simulink library "Copter_Library"  (Simulink 7.5)
settings: Solver=ode45  StartTime=0.0  StopTime=10.0  RelTol=1e-3
values from neighbouring files (symbols this model uses):
  phi0 = 0.15    [Quadrocopter_control_Driver.m]    (also in calc_stability.m = 0)
  r_phi0 = 0    [Quadrocopter_control_Driver.m]    (also in calc_stability.m)
  r_psi0 = 0    [Quadrocopter_control_Driver.m]    (also in calc_stability.m)
  r_theta0 = 0    [Quadrocopter_control_Driver.m]    (also in calc_stability.m)
  theta0 = 0.15    [Quadrocopter_control_Driver.m]    (also in calc_stability.m = 0)
  Ts = 0.01    [Reglerauslegung.m]    (also in Test_Reglerauslegung.m)
undefined symbols (not defined in the file or in its folder): boom, DiscIntNeverNeededParam, f1, f2, f3, f4, f5, g, I_x, I_y, I_z, m, speed, thrust, Ts_Opt
libraries: simulink x21, Copter_Library x17, vrlib x7, dspobslib x4, dspinverses x3, Control_lib x2
(part 1 of 3)
settings Model: Creator=robert  LastModifiedBy=Anonymos

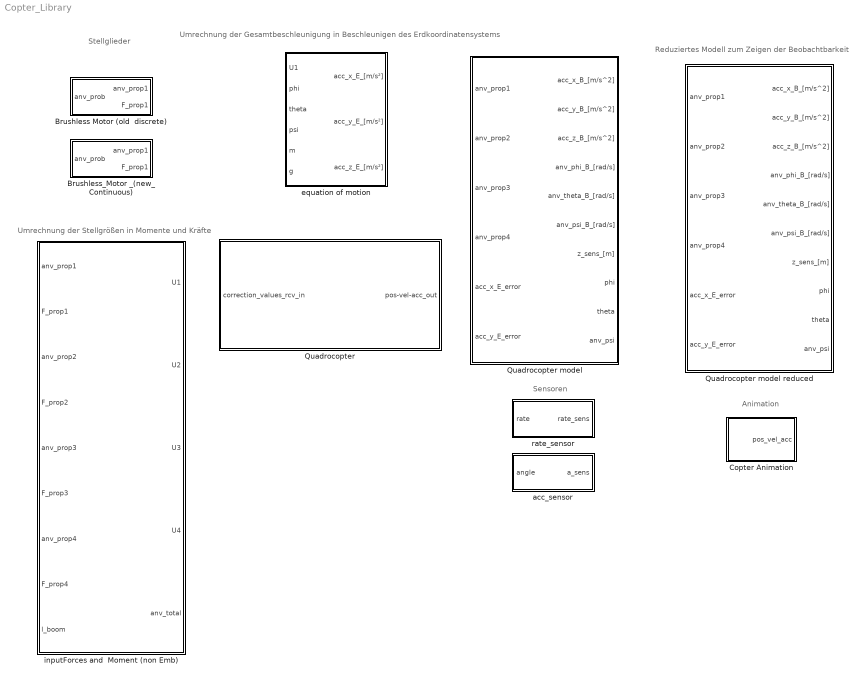
== system Copter_Library ==
  note: Sensoren
  note: Animation
  note: Umrechnung der Gesamtbeschleunigung in
      | Beschleunigen des Erdkoordinatensystems
  note: Stellglieder
  note: Umrechnung der Stellgrößen
      | in Momente und Kräfte
  note: Reduziertes Modell zum Zeigen der
      | Beobachtbarkeit
  Brushless Motor (old  discrete) : Subsystem
  Brushless_Motor _(new_Continuous) : Subsystem  mask{M_error=0.99}
      mask prompts: M_error "Motor-Force pitch error [1 = no error, 0.9 = 10% negativ error, 1.1 = 10% positive error]:"
  Copter Animation : Subsystem  mask(Quadrocopter Animation){AXES=[-100 100 -100 100 0 100], T_INT=1/25, K_VAR=Feste Position, K_POS=[10 0 2], K_ANGLE=27, A_ON=on, u_phi=on, u_theta=on, u_psi=on, u_x=on, u_y=on, u_z=off}
      mask prompts: AXES "Achsen Grenzen [xmin xmax ymin ymax zmin zmax]"; T_INT "Zeitintervall zwischen Aktualisierungen [s]:"; K_VAR "Kamera Art:"; K_POS "Ort der Kamera [xc yc zc]:"; K_ANGLE "Öffnungswinkel der Kamera [Grad]:"; A_ON "Animation Einschalten:"; u_phi "Use Input phi:"; u_theta "Use Input theta:"; u_psi "Use Input psi:"; u_x "Use Input x:"; u_y "Use Input y:"; u_z "Use Input z:"
      mask help: Erstellt eine 3-D animierte Ansicht eines Quadrocopters.
      mask init:
      | Config.axes = AXES;
      | Config.update = T_INT;
      | Config.camera_view = K_VAR;
      | Config.camera_pos = K_POS;
      | Config.view = K_ANGLE;
      | Config.Animenable = A_ON;
      | Config.phi = u_phi;
      | Config.theta = u_theta;
      | Config.psi = u_psi;
      | Config.x = u_x;
      | Config.y = u_y;
      | Config.z = u_z;
      mask Help:
      | <p>Dieser Block erstellt ein 3 dimensionales Fenster eines Quadrocopters.
      | 
      | <p><H4>Block Eingänge</H4>
      | Der Eingangsvektor bestehend aus:
      | <ul>
      | <li>X-Koordinate - Ort bezogen auf die X-Achse
      | <li>Y-Koordinate - Ort bezogen auf die Y-Achse
      | <li>Z-Koordinate - Ort bezogen auf die Z-Achse
      | <li>Psi - Yaw Drehung um die Z-Achse
      | <li>Phi - Roll Drehen um die Achse in Flugrichtung
      | <li>theta - pitch Neigung in Flugrichtung nach oben bzw. unten
      | </ul></p>
      mask StyleString: edit,edit,popup(Feste Position|Frei bewegbar),edit,edit,checkbox,checkbox,checkbox,checkbox,checkbox,checkbox,checkbox
  Quadrocopter : Subsystem
  Quadrocopter model : Subsystem
  Quadrocopter model reduced : Subsystem
  acc_sensor : Subsystem  mask{lsb_per_g=g/340, direction=1}
      mask prompts: lsb_per_g "Auflösung[LSB/g]:(g = Erdbeschleunigung)"; direction "Direction[-1 ... 1]:"
      mask init:
      | LSB_per_g = lsb_per_g;
      | Direction = direction;
  equation of motion : Subsystem
  inputForces and  Moment (non Emb) : Subsystem
  rate_sensor : Subsystem  mask{resolution=0.01423597337917052316100312926969, offset=505, direction=1}
      mask prompts: resolution "Resolution [(rad/sec)/LSB)]:"; offset "Offset [LSB]:"; direction "Direction [-1 ... 1]"
      mask init:
      | Resolution = resolution;
      | Offset = offset;
      | Direction = direction;

== system Copter_Library/Brushless Motor (old  discrete) ==
  note: Gain of BLDC1
  note: Kraft in Drehzahl umrechnen
  note: Registerwert in Kraft umsetzten
  note: Kraft verzögert, aber Drehzahl nicht ?
  anv_prob : Inport  OutDataType=fixdt(1, 16)  OutScaling=2^0
  Discrete Transfer Fcn : DiscreteTransferFcn  Numerator=[0.05]  Denominator=[1 -0.95]  SampleTime=Ts
  Gain6 : Gain  ParameterDataType=fixdt(1, 16)  ParameterScaling=2^0  OutDataType=fixdt(1, 16)  OutScaling=2^0
  setpoint_thrust_prop1 : Lookup  InputValues=[0 40 175]  Table=[0 500 4500]./1000  LookUpMeth=Interpolation-Use End Values  OutDataType=fixdt(1, 16)  OutScaling=2^0
  thrust_speed_prop1 : Lookup  InputValues=thrust  Table=speed  LookUpMeth=Interpolation-Use End Values  OutDataType=fixdt(1, 16)  OutScaling=2^0
  anv_prop1 : Outport  OutDataType=fixdt(1, 16)  OutScaling=2^0
  F_prop1 : Outport  Port=2  OutDataType=fixdt(1, 16)  OutScaling=2^0
  wires:
  anv_prob/1 -> setpoint_thrust_prop1/1
  Discrete Transfer Fcn/1 -> Gain6/1
  Gain6/1 -> F_prop1/1
  thrust_speed_prop1/1 -> anv_prop1/1
  setpoint_thrust_prop1/1 -> thrust_speed_prop1/1, Discrete Transfer Fcn/1

== system Copter_Library/Brushless_Motor _(new_Continuous) ==
  note: Gain of BLDC
  note: Kraft in Drehzahl umrechnen
  note: Registerwert in Kraft umsetzten
  note: Verrzögerung des Kraft
  note: Brushless Motor (new Continuous)
  anv_prob : Inport  OutDataType=fixdt(1, 16)  OutScaling=2^0
  Data Type Conversion : DataTypeConversion  OutDataTypeMode=double  OutDataType=fixdt(1, 16)  OutScaling=2^0  OutDataTypeStr=double
  Gain6 : Gain  Gain=M_error  ParameterDataType=fixdt(1, 16)  ParameterScaling=2^0  OutDataType=fixdt(1, 16)  OutScaling=2^0
  Motor_Delay : TransferFcn  Denominator=[0.001 1]  ContinuousStateAttributes='Motor_Delay'
  Saturation : Saturate  UpperLimit=255  LowerLimit=0  OutDataType=fixdt(1, 16)  OutScaling=2^0
  setpoint_thrust_prop : Lookup  InputValues=[0 40 175]  Table=[0 500 4500]./1000  LookUpMeth=Interpolation-Use End Values  OutDataType=fixdt(1, 16)  OutScaling=2^0
  thrust_speed_prop : Lookup  InputValues=thrust  Table=speed  LookUpMeth=Interpolation-Use End Values  OutDataType=fixdt(1, 16)  OutScaling=2^0
  anv_prop1 : Outport  OutDataType=fixdt(1, 16)  OutScaling=2^0
  F_prop1 : Outport  Port=2  OutDataType=fixdt(1, 16)  OutScaling=2^0
  wires:
  setpoint_thrust_prop/1 -> Motor_Delay/1
  Saturation/1 -> Data Type Conversion/1
  anv_prob/1 -> Saturation/1
  Data Type Conversion/1 -> setpoint_thrust_prop/1
  Motor_Delay/1 -> Gain6/1
  Gain6/1 -> F_prop1/1, thrust_speed_prop/1
  thrust_speed_prop/1 -> anv_prop1/1

== system Copter_Library/Copter Animation ==
  pos_vel_acc : Inport  PortDimensions=19  OutDataType=sfix(16)  OutScaling=2^0
  S-Function : S-Function  FunctionName=Copter_Animation  Parameters=Config  EnableBusSupport=off
  Selector2 : Selector  InputPortWidth=19  IndexOptions=Index vector (dialog)  Indices=[1 2 3 4 5 6]  OutputSizes=1
  wires:
  Selector2/1 -> S-Function/1
  pos_vel_acc/1 -> Selector2/1

== system Copter_Library/Quadrocopter ==
  note: pos-vel-acc: [x, y, z, phi(roll), theta(pitch), psi(yaw), vx, vy, vz,rphi(roll rate), rtheta(pitch rate), rpsi(yaw rate),ax, ay, az,aphi(roll rate), atheta(pitch rate), apsi(yaw rate)]
  correction_values_rcv_in : Inport
  Analysis Lab : Subsystem
      mask Display: image(imresize(imread('DecoImg/Lab.jpg'),0.12), 'center');
  Control : Subsystem
      mask Display: image(imresize(imread('DecoImg/Control.jpg'),0.2), 'center');
  Dynamics : Subsystem
      mask Display: image(imresize(imread('DecoImg/Dynamics.jpg'),0.2), 'center');
  Environmetal influences : Subsystem
      mask Display: image(imresize(imread('DecoImg/Environment.jpg'),0.2), 'center');
  Remote Control : Subsystem
      mask Display: image(imresize(imread('DecoImg/RemoteControl.jpg'),0.4), 'center');
  Sensors : Subsystem
      mask Display: image(imresize(imread('DecoImg/Sensors.jpg'),0.1), 'center');
  pos-vel-acc_out : Outport
  wires:
  Control/1(Motors) -> Dynamics/2(Motors)
  Dynamics/1(pos-vel-acc) -> Analysis Lab/1(pos-vel-acc_in), Sensors/1(pos-vel-acc), pos-vel-acc_out/1  "pos-vel-acc"
  Sensors/2(IMU) -> Control/3(IMU)  "ax  ay  rphi  rtheta rpsi"
  Remote Control/1(RC_out) -> Control/1(Task)  "phi(roll) theta(pitch) rpsi(yaw rate) T(thrust)"
  Sensors/1(height) -> Control/4(height)  "height"
  Sensors/3(correction) -> Control/2(correction)  "vx vy rpsi"
  Environmetal influences/1(vel_err) -> Dynamics/1(vel_errors)
  correction_values_rcv_in/1 -> Sensors/2(correction_values_rcv)

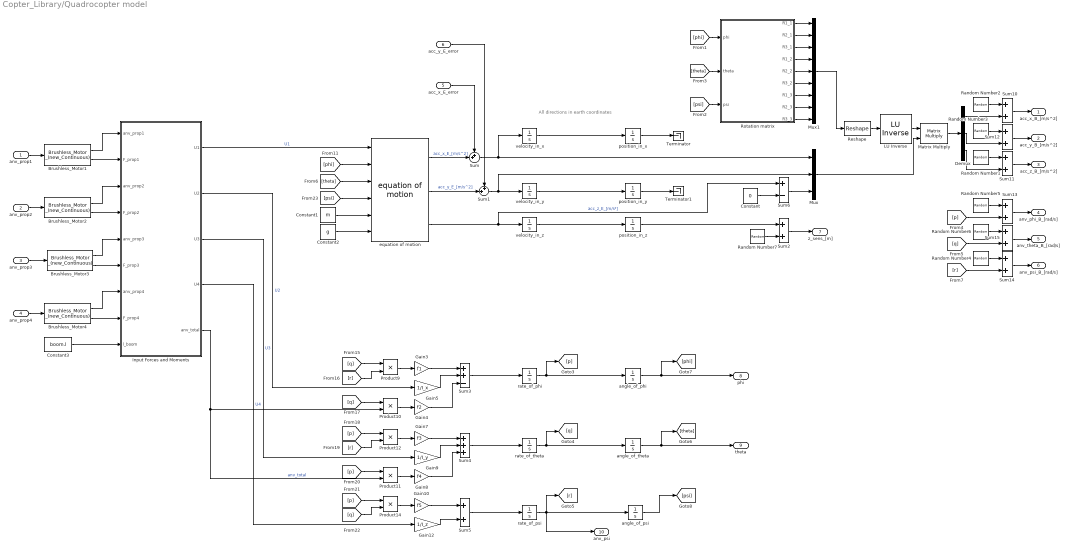
== system Copter_Library/Quadrocopter model ==
  note: All directions in earth coordinates
  anv_prop1 : Inport  OutDataType=fixdt(1, 16)  OutScaling=2^0
  anv_prop2 : Inport  Port=2  OutDataType=fixdt(1, 16)  OutScaling=2^0
  anv_prop3 : Inport  Port=3  OutDataType=fixdt(1, 16)  OutScaling=2^0
  anv_prop4 : Inport  Port=4  OutDataType=fixdt(1, 16)  OutScaling=2^0
  acc_x_E_error : Inport  Port=5  OutDataType=fixdt(1, 16)  OutScaling=2^0
  acc_y_E_error : Inport  Port=6  OutDataType=fixdt(1, 16)  OutScaling=2^0
  " LU Inverse" : dspinverses/ LU Inverse  SystemSampleTime=-1
  Brushless_Motor{1..4} (4 alike) : Copter_Library/Brushless_Motor _(new_Continuous)  SystemSampleTime=-1
  Constant : Constant  Value=0  OutDataType=fixdt(1, 16)  OutScaling=2^0  SampleTime=Ts
  Constant1 : Constant  Value=m  OutDataType=fixdt(1, 16)  OutScaling=2^0  SampleTime=Ts
  Constant2 : Constant  Value=g  OutDataType=fixdt(1, 16)  OutScaling=2^0  SampleTime=Ts
  Constant3 : Constant  Value=boom.l  OutDataType=fixdt(1, 16)  OutScaling=2^0
  Demux : Demux  Outputs=3
  Gain10 : Gain  Gain=f5  ParameterDataType=fixdt(1, 16)  ParameterScaling=2^0  OutDataType=fixdt(1, 16)  OutScaling=2^0
  Gain12 : Gain  Gain=1/I_z  ParameterDataType=fixdt(1, 16)  ParameterScaling=2^0  OutDataType=fixdt(1, 16)  OutScaling=2^0
  Gain3 : Gain  Gain=f1  ParameterDataType=fixdt(1, 16)  ParameterScaling=2^0  OutDataType=fixdt(1, 16)  OutScaling=2^0
  Gain4 : Gain  Gain=f2  ParameterDataType=fixdt(1, 16)  ParameterScaling=2^0  OutDataType=fixdt(1, 16)  OutScaling=2^0
  Gain5 : Gain  Gain=1/I_x  ParameterDataType=fixdt(1, 16)  ParameterScaling=2^0  OutDataType=fixdt(1, 16)  OutScaling=2^0
  Gain7 : Gain  Gain=f3  ParameterDataType=fixdt(1, 16)  ParameterScaling=2^0  OutDataType=fixdt(1, 16)  OutScaling=2^0
  Gain8 : Gain  Gain=f4  ParameterDataType=fixdt(1, 16)  ParameterScaling=2^0  OutDataType=fixdt(1, 16)  OutScaling=2^0
  Gain9 : Gain  Gain=1/I_y  ParameterDataType=fixdt(1, 16)  ParameterScaling=2^0  OutDataType=fixdt(1, 16)  OutScaling=2^0
  Input Forces and Moments : Stateflow chart  TreatAsAtomicUnit=on
  Matrix Multiply : Product  Multiplication=Matrix(*)  OutDataType=sfix(16)  OutScaling=2^0
  Mux : Mux  Inputs=3
  Mux1 : Mux  Inputs=9
  Product{9..12,14} (5 alike) : Product  OutDataType=fixdt(1, 16)  OutScaling=2^0  RndMeth=Zero
  Random Number{1..7} (7 alike) : RandomNumber  Variance=0  SampleTime=Ts
  Reshape : Reshape  OutputDimensionality=Customize  OutputDimensions=[3,3]
  Rotation matrix : Stateflow chart  TreatAsAtomicUnit=on
  Sum : Sum  Inputs=++|  OutDataType=fixdt(1, 16)  OutScaling=2^0
  Sum1 : Sum  Inputs=++|  OutDataType=fixdt(1, 16)  OutScaling=2^0
  Sum{2,5,10..15} (8 alike) : Sum  OutDataType=fixdt(1, 16)  OutScaling=2^0
  Sum3 : Sum  Inputs=++-  OutDataType=fixdt(1, 16)  OutScaling=2^0
  Sum4 : Sum  Inputs=+++  OutDataType=fixdt(1, 16)  OutScaling=2^0
  Sum6 : Sum  Inputs=+-  OutDataType=fixdt(1, 16)  OutScaling=2^0
  Terminator : Terminator
  Terminator1 : Terminator
  angle_of_phi : Integrator
  angle_of_psi : Integrator
  angle_of_theta : Integrator
  equation of motion : Copter_Library/equation of motion  SystemSampleTime=-1
  position_in_x : Integrator
  position_in_y : Integrator
  position_in_z : Integrator
  rate_of_phi : Integrator
  rate_of_psi : Integrator
  rate_of_theta : Integrator
  velocity_in_x : Integrator
  velocity_in_y : Integrator
  velocity_in_z : Integrator
  acc_x_B_[m/s^2] : Outport  OutDataType=fixdt(1, 16)  OutScaling=2^0
  acc_y_B_[m/s^2] : Outport  Port=2  OutDataType=fixdt(1, 16)  OutScaling=2^0
  acc_z_B_[m/s^2] : Outport  Port=3  OutDataType=fixdt(1, 16)  OutScaling=2^0
  anv_phi_B_[rad/s] : Outport  Port=4  OutDataType=fixdt(1, 16)  OutScaling=2^0
  anv_theta_B_[rad/s] : Outport  Port=5  OutDataType=fixdt(1, 16)  OutScaling=2^0
  anv_psi_B_[rad/s] : Outport  Port=6  OutDataType=fixdt(1, 16)  OutScaling=2^0
  z_sens_[m] : Outport  Port=7  OutDataType=fixdt(1, 16)  OutScaling=2^0
  phi : Outport  Port=8  OutDataType=fixdt(1, 16)  OutScaling=2^0
  theta : Outport  Port=9  OutDataType=fixdt(1, 16)  OutScaling=2^0
  anv_psi : Outport  Port=10  OutDataType=fixdt(1, 16)  OutScaling=2^0
  wires:
  Sum14/1 -> anv_psi_B_[rad/s]/1
  Sum15/1 -> anv_theta_B_[rad/s]/1
  Sum13/1 -> anv_phi_B_[rad/s]/1
  [q] -> Sum15/2
  Random Number6/1 -> Sum15/1
  [r] -> Sum14/2
  Random Number4/1 -> Sum14/1
  [p] -> Sum13/2
  Random Number5/1 -> Sum13/1
  Sum11/1 -> acc_z_B_[m/s^2]/1
  Sum12/1 -> acc_y_B_[m/s^2]/1
  Sum10/1 -> acc_x_B_[m/s^2]/1
  Demux/2 -> Sum12/2
  Random Number3/1 -> Sum12/1
  Demux/3 -> Sum11/2
  Random Number1/1 -> Sum11/1
  Demux/1 -> Sum10/2
  Random Number2/1 -> Sum10/1
  Matrix Multiply/1 -> Demux/1
  anv_prop3/1 -> Brushless_Motor3/1
  anv_prop4/1 -> Brushless_Motor4/1
  Reshape/1 -> " LU Inverse"/1
  Mux/1 -> Matrix Multiply/2
  Mux1/1 -> Reshape/1
  Rotation matrix/9(R3_3) -> Mux1/9
  Rotation matrix/8(R2_3) -> Mux1/8
  Rotation matrix/7(R1_3) -> Mux1/7
  Rotation matrix/6(R3_2) -> Mux1/6
  Rotation matrix/5(R2_2) -> Mux1/5
  Rotation matrix/4(R1_2) -> Mux1/4
  Rotation matrix/3(R3_1) -> Mux1/3
  Rotation matrix/2(R2_1) -> Mux1/2
  Rotation matrix/1(R1_1) -> Mux1/1
  [psi] -> Rotation matrix/3(psi)
  [theta] -> Rotation matrix/2(theta)
  [phi] -> Rotation matrix/1(phi)
  anv_prop2/1 -> Brushless_Motor2/1
  anv_prop1/1 -> Brushless_Motor1/1
  velocity_in_x/1 -> position_in_x/1
  velocity_in_y/1 -> position_in_y/1
  velocity_in_z/1 -> position_in_z/1
  Constant3/1 -> Input Forces and Moments/9(l_boom)
  Sum5/1 -> rate_of_psi/1
  Input Forces and Moments/4(U4) -> Gain12/1  "U4"
  Gain12/1 -> Sum5/2
  Gain10/1 -> Sum5/1
  Product14/1 -> Gain10/1
  [q] -> Product14/2
  [p] -> Product14/1
  Sum4/1 -> rate_of_theta/1
  Input Forces and Moments/3(U3) -> Gain9/1  "U3"
  Gain8/1 -> Sum4/3
  Gain9/1 -> Sum4/2
  Product11/1 -> Gain8/1
  [p] -> Product11/1
  Gain7/1 -> Sum4/1
  Product12/1 -> Gain7/1
  [r] -> Product12/2
  [p] -> Product12/1
  Input Forces and Moments/1(U1) -> equation of motion/1  "U1"
  Sum3/1 -> rate_of_phi/1
  Gain4/1 -> Sum3/3
  Gain5/1 -> Sum3/2
  Input Forces and Moments/2(U2) -> Gain5/1  "U2"
  Product10/1 -> Gain4/1
  [q] -> Product10/1
  Gain3/1 -> Sum3/1
  Product9/1 -> Gain3/1
  [r] -> Product9/2
  [q] -> Product9/1
  Input Forces and Moments/5(anv_total) -> Product11/2, Product10/2  "anv_total"
  angle_of_phi/1 -> [phi], phi/1
  angle_of_theta/1 -> [theta], theta/1
  angle_of_psi/1 -> [psi]
  rate_of_phi/1 -> [p], angle_of_phi/1
  rate_of_theta/1 -> angle_of_theta/1, [q]
  rate_of_psi/1 -> anv_psi/1, angle_of_psi/1, [r]
  Constant/1 -> Sum6/2
  Sum6/1 -> Mux/3
  " LU Inverse"/1 -> Matrix Multiply/1
  Brushless_Motor1/1 -> Input Forces and Moments/1(anv_prop1)
  Brushless_Motor1/2 -> Input Forces and Moments/2(F_prop1)
  Brushless_Motor2/1 -> Input Forces and Moments/3(anv_prop2)
  Brushless_Motor2/2 -> Input Forces and Moments/4(F_prop2)
  Brushless_Motor3/1 -> Input Forces and Moments/5(anv_prop3)
  Brushless_Motor3/2 -> Input Forces and Moments/6(F_prop3)
  Brushless_Motor4/1 -> Input Forces and Moments/7(anv_prop4)
  Brushless_Motor4/2 -> Input Forces and Moments/8(F_prop4)
  [phi] -> equation of motion/2
  [theta] -> equation of motion/3
  [psi] -> equation of motion/4
  Constant1/1 -> equation of motion/5
  Constant2/1 -> equation of motion/6
  equation of motion/3 -> velocity_in_z/1, Sum6/1  "acc_z_E_[m/s²]"
  position_in_x/1 -> Terminator/1
  position_in_y/1 -> Terminator1/1
  Sum1/1 -> velocity_in_y/1, Mux/2
  equation of motion/2 -> Sum1/2  "acc_y_E_[m/s^2]"
  equation of motion/1 -> Sum/2  "acc_x_E_[m/s^2]"
  Sum/1 -> Mux/1, velocity_in_x/1
  acc_x_E_error/1 -> Sum/1
  acc_y_E_error/1 -> Sum1/1
  position_in_z/1 -> Sum2/1
  Sum2/1 -> z_sens_[m]/1
  Random Number7/1 -> Sum2/2

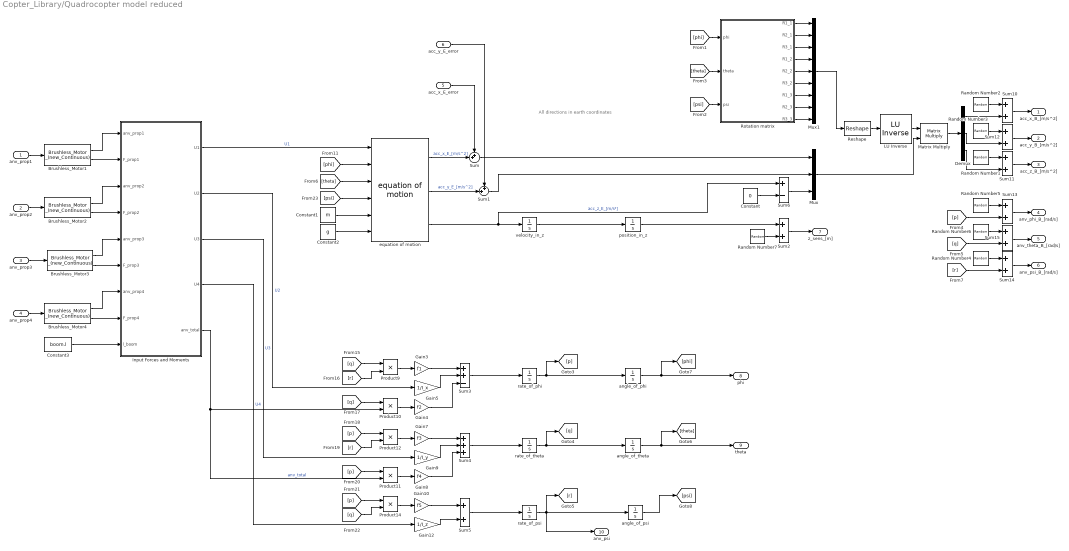
== system Copter_Library/Quadrocopter model reduced ==
  note: All directions in earth coordinates
  anv_prop1 : Inport  OutDataType=fixdt(1, 16)  OutScaling=2^0
  anv_prop2 : Inport  Port=2  OutDataType=fixdt(1, 16)  OutScaling=2^0
  anv_prop3 : Inport  Port=3  OutDataType=fixdt(1, 16)  OutScaling=2^0
  anv_prop4 : Inport  Port=4  OutDataType=fixdt(1, 16)  OutScaling=2^0
  acc_x_E_error : Inport  Port=5  OutDataType=fixdt(1, 16)  OutScaling=2^0
  acc_y_E_error : Inport  Port=6  OutDataType=fixdt(1, 16)  OutScaling=2^0
  " LU Inverse" : dspinverses/ LU Inverse  SystemSampleTime=-1
  Brushless_Motor{1..4} (4 alike) : Copter_Library/Brushless_Motor _(new_Continuous)  SystemSampleTime=-1
  Constant : Constant  Value=0  OutDataType=fixdt(1, 16)  OutScaling=2^0  SampleTime=Ts
  Constant1 : Constant  Value=m  OutDataType=fixdt(1, 16)  OutScaling=2^0  SampleTime=Ts
  Constant2 : Constant  Value=g  OutDataType=fixdt(1, 16)  OutScaling=2^0  SampleTime=Ts
  Constant3 : Constant  Value=boom.l  OutDataType=fixdt(1, 16)  OutScaling=2^0
  Demux : Demux  Outputs=3
  Gain10 : Gain  Gain=f5  ParameterDataType=fixdt(1, 16)  ParameterScaling=2^0  OutDataType=fixdt(1, 16)  OutScaling=2^0
  Gain12 : Gain  Gain=1/I_z  ParameterDataType=fixdt(1, 16)  ParameterScaling=2^0  OutDataType=fixdt(1, 16)  OutScaling=2^0
  Gain3 : Gain  Gain=f1  ParameterDataType=fixdt(1, 16)  ParameterScaling=2^0  OutDataType=fixdt(1, 16)  OutScaling=2^0
  Gain4 : Gain  Gain=f2  ParameterDataType=fixdt(1, 16)  ParameterScaling=2^0  OutDataType=fixdt(1, 16)  OutScaling=2^0
  Gain5 : Gain  Gain=1/I_x  ParameterDataType=fixdt(1, 16)  ParameterScaling=2^0  OutDataType=fixdt(1, 16)  OutScaling=2^0
  Gain7 : Gain  Gain=f3  ParameterDataType=fixdt(1, 16)  ParameterScaling=2^0  OutDataType=fixdt(1, 16)  OutScaling=2^0
  Gain8 : Gain  Gain=f4  ParameterDataType=fixdt(1, 16)  ParameterScaling=2^0  OutDataType=fixdt(1, 16)  OutScaling=2^0
  Gain9 : Gain  Gain=1/I_y  ParameterDataType=fixdt(1, 16)  ParameterScaling=2^0  OutDataType=fixdt(1, 16)  OutScaling=2^0
  Input Forces and Moments : Stateflow chart  TreatAsAtomicUnit=on
  Matrix Multiply : Product  Multiplication=Matrix(*)  OutDataType=sfix(16)  OutScaling=2^0
  Mux : Mux  Inputs=3
  Mux1 : Mux  Inputs=9
  Product{9..12,14} (5 alike) : Product  OutDataType=fixdt(1, 16)  OutScaling=2^0  RndMeth=Zero
  Random Number{1..7} (7 alike) : RandomNumber  Variance=0  SampleTime=Ts
  Reshape : Reshape  OutputDimensionality=Customize  OutputDimensions=[3,3]
  Rotation matrix : Stateflow chart  TreatAsAtomicUnit=on
  Sum : Sum  Inputs=++|  OutDataType=fixdt(1, 16)  OutScaling=2^0
  Sum1 : Sum  Inputs=++|  OutDataType=fixdt(1, 16)  OutScaling=2^0
  Sum{2,5,10..15} (8 alike) : Sum  OutDataType=fixdt(1, 16)  OutScaling=2^0
  Sum3 : Sum  Inputs=++-  OutDataType=fixdt(1, 16)  OutScaling=2^0
  Sum4 : Sum  Inputs=+++  OutDataType=fixdt(1, 16)  OutScaling=2^0
  Sum6 : Sum  Inputs=+-  OutDataType=fixdt(1, 16)  OutScaling=2^0
  angle_of_phi : Integrator
  angle_of_psi : Integrator
  angle_of_theta : Integrator
  equation of motion : Copter_Library/equation of motion  SystemSampleTime=-1
  position_in_z : Integrator
  rate_of_phi : Integrator
  rate_of_psi : Integrator
  rate_of_theta : Integrator
  velocity_in_z : Integrator
  acc_x_B_[m/s^2] : Outport  OutDataType=fixdt(1, 16)  OutScaling=2^0
  acc_y_B_[m/s^2] : Outport  Port=2  OutDataType=fixdt(1, 16)  OutScaling=2^0
  acc_z_B_[m/s^2] : Outport  Port=3  OutDataType=fixdt(1, 16)  OutScaling=2^0
  anv_phi_B_[rad/s] : Outport  Port=4  OutDataType=fixdt(1, 16)  OutScaling=2^0
  anv_theta_B_[rad/s] : Outport  Port=5  OutDataType=fixdt(1, 16)  OutScaling=2^0
  anv_psi_B_[rad/s] : Outport  Port=6  OutDataType=fixdt(1, 16)  OutScaling=2^0
  z_sens_[m] : Outport  Port=7  OutDataType=fixdt(1, 16)  OutScaling=2^0
  phi : Outport  Port=8  OutDataType=fixdt(1, 16)  OutScaling=2^0
  theta : Outport  Port=9  OutDataType=fixdt(1, 16)  OutScaling=2^0
  anv_psi : Outport  Port=10  OutDataType=fixdt(1, 16)  OutScaling=2^0
  wires:
  Sum14/1 -> anv_psi_B_[rad/s]/1
  Sum15/1 -> anv_theta_B_[rad/s]/1
  Sum13/1 -> anv_phi_B_[rad/s]/1
  [q] -> Sum15/2
  Random Number6/1 -> Sum15/1
  [r] -> Sum14/2
  Random Number4/1 -> Sum14/1
  [p] -> Sum13/2
  Random Number5/1 -> Sum13/1
  Sum11/1 -> acc_z_B_[m/s^2]/1
  Sum12/1 -> acc_y_B_[m/s^2]/1
  Sum10/1 -> acc_x_B_[m/s^2]/1
  Demux/2 -> Sum12/2
  Random Number3/1 -> Sum12/1
  Demux/3 -> Sum11/2
  Random Number1/1 -> Sum11/1
  Demux/1 -> Sum10/2
  Random Number2/1 -> Sum10/1
  Matrix Multiply/1 -> Demux/1
  anv_prop3/1 -> Brushless_Motor3/1
  anv_prop4/1 -> Brushless_Motor4/1
  Reshape/1 -> " LU Inverse"/1
  Mux/1 -> Matrix Multiply/2
  Mux1/1 -> Reshape/1
  Rotation matrix/9(R3_3) -> Mux1/9
  Rotation matrix/8(R2_3) -> Mux1/8
  Rotation matrix/7(R1_3) -> Mux1/7
  Rotation matrix/6(R3_2) -> Mux1/6
  Rotation matrix/5(R2_2) -> Mux1/5
  Rotation matrix/4(R1_2) -> Mux1/4
  Rotation matrix/3(R3_1) -> Mux1/3
  Rotation matrix/2(R2_1) -> Mux1/2
  Rotation matrix/1(R1_1) -> Mux1/1
  [psi] -> Rotation matrix/3(psi)
  [theta] -> Rotation matrix/2(theta)
  [phi] -> Rotation matrix/1(phi)
  anv_prop2/1 -> Brushless_Motor2/1
  anv_prop1/1 -> Brushless_Motor1/1
  velocity_in_z/1 -> position_in_z/1
  Constant3/1 -> Input Forces and Moments/9(l_boom)
  Sum5/1 -> rate_of_psi/1
  Input Forces and Moments/4(U4) -> Gain12/1  "U4"
  Gain12/1 -> Sum5/2
  Gain10/1 -> Sum5/1
  Product14/1 -> Gain10/1
  [q] -> Product14/2
  [p] -> Product14/1
  Sum4/1 -> rate_of_theta/1
  Input Forces and Moments/3(U3) -> Gain9/1  "U3"
  Gain8/1 -> Sum4/3
  Gain9/1 -> Sum4/2
  Product11/1 -> Gain8/1
  [p] -> Product11/1
  Gain7/1 -> Sum4/1
  Product12/1 -> Gain7/1
  [r] -> Product12/2
  [p] -> Product12/1
  Input Forces and Moments/1(U1) -> equation of motion/1  "U1"
  Sum3/1 -> rate_of_phi/1
  Gain4/1 -> Sum3/3
  Gain5/1 -> Sum3/2
  Input Forces and Moments/2(U2) -> Gain5/1  "U2"
  Product10/1 -> Gain4/1
  [q] -> Product10/1
  Gain3/1 -> Sum3/1
  Product9/1 -> Gain3/1
  [r] -> Product9/2
  [q] -> Product9/1
  Input Forces and Moments/5(anv_total) -> Product11/2, Product10/2  "anv_total"
  angle_of_phi/1 -> [phi], phi/1
  angle_of_theta/1 -> [theta], theta/1
  angle_of_psi/1 -> [psi]
  rate_of_phi/1 -> [p], angle_of_phi/1
  rate_of_theta/1 -> angle_of_theta/1, [q]
  rate_of_psi/1 -> anv_psi/1, angle_of_psi/1, [r]
  Constant/1 -> Sum6/2
  Sum6/1 -> Mux/3
  " LU Inverse"/1 -> Matrix Multiply/1
  Brushless_Motor1/1 -> Input Forces and Moments/1(anv_prop1)
  Brushless_Motor1/2 -> Input Forces and Moments/2(F_prop1)
  Brushless_Motor2/1 -> Input Forces and Moments/3(anv_prop2)
  Brushless_Motor2/2 -> Input Forces and Moments/4(F_prop2)
  Brushless_Motor3/1 -> Input Forces and Moments/5(anv_prop3)
  Brushless_Motor3/2 -> Input Forces and Moments/6(F_prop3)
  Brushless_Motor4/1 -> Input Forces and Moments/7(anv_prop4)
  Brushless_Motor4/2 -> Input Forces and Moments/8(F_prop4)
  [phi] -> equation of motion/2
  [theta] -> equation of motion/3
  [psi] -> equation of motion/4
  Constant1/1 -> equation of motion/5
  Constant2/1 -> equation of motion/6
  equation of motion/3 -> velocity_in_z/1, Sum6/1  "acc_z_E_[m/s²]"
  Sum1/1 -> Mux/2
  equation of motion/2 -> Sum1/2  "acc_y_E_[m/s^2]"
  equation of motion/1 -> Sum/2  "acc_x_E_[m/s^2]"
  Sum/1 -> Mux/1
  acc_x_E_error/1 -> Sum/1
  acc_y_E_error/1 -> Sum1/1
  position_in_z/1 -> Sum2/1
  Sum2/1 -> z_sens_[m]/1
  Random Number7/1 -> Sum2/2

== system Copter_Library/acc_sensor ==
  note: inverted like in the real copter
  angle : Inport  OutDataType=fixdt(1, 16)  OutScaling=2^0
  Gain1 : Gain  Gain=Direction  ParameterDataType=fixdt(1, 16)  ParameterScaling=2^0  OutDataType=fixdt(1, 16)  OutScaling=2^0
  Gain19 : Gain  Gain=-1/LSB_per_g  ParameterDataType=fixdt(1, 16)  ParameterScaling=2^0  OutDataType=fixdt(1, 16)  OutScaling=2^0
  Gain22 : Gain  Gain=g  ParameterDataType=fixdt(1, 16)  ParameterScaling=2^0  OutDataType=fixdt(1, 16)  OutScaling=2^0
  Quantizer3 : Quantizer  QuantizationInterval=LSB_per_g  SampleTime=Ts
  Random Number2 : RandomNumber  Variance=0.0003  Seed=4564  SampleTime=0.01
  Sum12 : Sum  OutDataType=fixdt(1, 16)  OutScaling=2^0
  Trigonometric Function : Trigonometry
  a_sens : Outport  OutDataType=fixdt(1, 16)  OutScaling=2^0
  wires:
  Random Number2/1 -> Sum12/1
  Sum12/1 -> Quantizer3/1
  Trigonometric Function/1 -> Gain22/1
  Gain22/1 -> Sum12/2
  Quantizer3/1 -> Gain19/1
  angle/1 -> Trigonometric Function/1
  Gain19/1 -> Gain1/1
  Gain1/1 -> a_sens/1

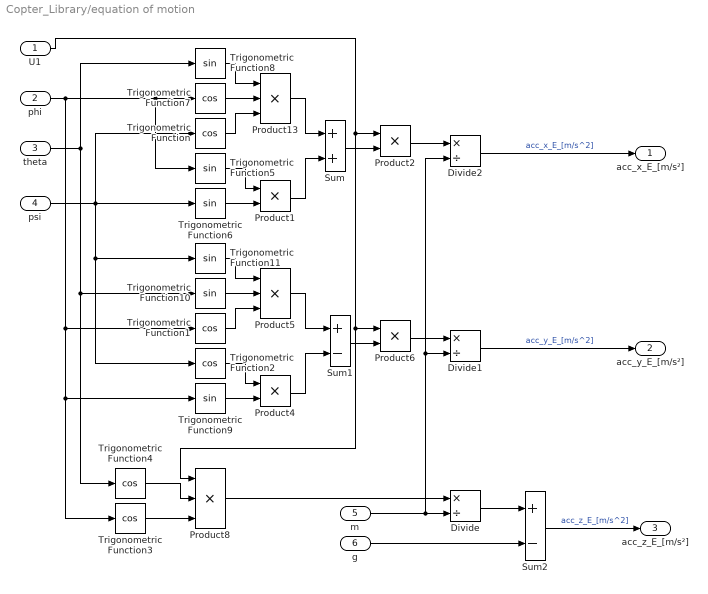
== system Copter_Library/equation of motion ==
  U1 : Inport  OutDataType=fixdt(1, 16)  OutScaling=2^0
  phi : Inport  Port=2  OutDataType=fixdt(1, 16)  OutScaling=2^0
  theta : Inport  Port=3  OutDataType=fixdt(1, 16)  OutScaling=2^0
  psi : Inport  Port=4  OutDataType=fixdt(1, 16)  OutScaling=2^0
  m : Inport  Port=5  OutDataType=fixdt(1, 16)  OutScaling=2^0
  g : Inport  Port=6  OutDataType=fixdt(1, 16)  OutScaling=2^0
  Divide : Product  Inputs=*/  OutDataType=fixdt(1, 16)  OutScaling=2^-10
  Divide1 : Product  Inputs=*/  OutDataType=fixdt(1, 16)  OutScaling=2^-10
  Divide2 : Product  Inputs=*/  OutDataType=fixdt(1, 16)  OutScaling=2^-10
  Product{1..2,4,6} (4 alike) : Product  OutDataType=fixdt(1, 16)  OutScaling=2^0  RndMeth=Zero
  Product13 : Product  Inputs=3  OutDataType=fixdt(1, 16)  OutScaling=2^0  RndMeth=Zero
  Product5 : Product  Inputs=3  OutDataType=fixdt(1, 16)  OutScaling=2^0  RndMeth=Zero
  Product8 : Product  Inputs=3  OutDataType=fixdt(1, 16)  OutScaling=2^0  RndMeth=Zero
  Sum : Sum  OutDataType=fixdt(1, 16)  OutScaling=2^0
  Sum1 : Sum  Inputs=+-  OutDataType=fixdt(1, 16)  OutScaling=2^0
  Sum2 : Sum  Inputs=+-  OutDataType=fixdt(1, 16)  OutScaling=2^0
  Trigonometric Function{,1..4,7} (6 alike) : Trigonometry  Operator=cos
  Trigonometric Function{5..6,8..11} (6 alike) : Trigonometry
  acc_x_E_[m/s²] : Outport  OutDataType=fixdt(1, 16)  OutScaling=2^0
  acc_y_E_[m/s²] : Outport  Port=2  OutDataType=fixdt(1, 16)  OutScaling=2^0
  acc_z_E_[m/s²] : Outport  Port=3  OutDataType=fixdt(1, 16)  OutScaling=2^0
  wires:
  g/1 -> Sum2/2
  Trigonometric Function4/1 -> Product8/2
  Trigonometric Function3/1 -> Product8/3
  Divide/1 -> Sum2/1
  Divide2/1 -> acc_x_E_[m/s²]/1  "acc_x_E_[m/s^2]"
  Product6/1 -> Divide1/1
  Sum1/1 -> Product6/2
  Product5/1 -> Sum1/1
  Trigonometric Function1/1 -> Product5/3
  Trigonometric Function10/1 -> Product5/2
  Trigonometric Function11/1 -> Product5/1
  Product4/1 -> Sum1/2
  Trigonometric Function2/1 -> Product4/1
  Trigonometric Function9/1 -> Product4/2
  Product2/1 -> Divide2/1
  Sum/1 -> Product2/2
  Product13/1 -> Sum/1
  Trigonometric Function/1 -> Product13/3
  Trigonometric Function7/1 -> Product13/2
  Trigonometric Function8/1 -> Product13/1
  Product1/1 -> Sum/2
  Trigonometric Function5/1 -> Product1/1
  Trigonometric Function6/1 -> Product1/2
  psi/1 -> Trigonometric Function2/1, Trigonometric Function11/1, Trigonometric Function/1, Trigonometric Function6/1
  theta/1 -> Trigonometric Function10/1, Trigonometric Function4/1, Trigonometric Function8/1
  Divide1/1 -> acc_y_E_[m/s²]/1  "acc_y_E_[m/s^2]"
  phi/1 -> Trigonometric Function9/1, Trigonometric Function3/1, Trigonometric Function1/1, Trigonometric Function7/1, Trigonometric Function5/1
  Product8/1 -> Divide/1
  U1/1 -> Product8/1, Product6/1, Product2/1
  m/1 -> Divide/2, Divide1/2, Divide2/2
  Sum2/1 -> acc_z_E_[m/s²]/1  "acc_z_E_[m/s^2]"

== system Copter_Library/inputForces and  Moment (non Emb) ==
  anv_prop1 : Inport  OutDataType=fixdt(1, 16)  OutScaling=2^0
  F_prop1 : Inport  Port=2  OutDataType=fixdt(1, 16)  OutScaling=2^0
  anv_prop2 : Inport  Port=3  OutDataType=fixdt(1, 16)  OutScaling=2^0
  F_prop2 : Inport  Port=4  OutDataType=fixdt(1, 16)  OutScaling=2^0
  anv_prop3 : Inport  Port=5  OutDataType=fixdt(1, 16)  OutScaling=2^0
  F_prop3 : Inport  Port=6  OutDataType=fixdt(1, 16)  OutScaling=2^0
  anv_prop4 : Inport  Port=7  OutDataType=fixdt(1, 16)  OutScaling=2^0
  F_prop4 : Inport  Port=8  OutDataType=fixdt(1, 16)  OutScaling=2^0
  l_boom : Inport  Port=9  OutDataType=fixdt(1, 16)  OutScaling=2^0
  Product : Product  OutDataType=fixdt(1, 16)  OutScaling=2^0  RndMeth=Zero
  Product1 : Product  OutDataType=fixdt(1, 16)  OutScaling=2^0  RndMeth=Zero
  Product2 : Product  OutDataType=fixdt(1, 16)  OutScaling=2^0  RndMeth=Zero
  Sum : Sum  Inputs=+-+-  OutDataType=fixdt(1, 16)  OutScaling=2^0
  Sum1 : Sum  Inputs=++++  OutDataType=fixdt(1, 16)  OutScaling=2^0
  Sum2 : Sum  Inputs=+-+-  OutDataType=fixdt(1, 16)  OutScaling=2^0
  Sum3 : Sum  Inputs=-+  OutDataType=fixdt(1, 16)  OutScaling=2^0
  Sum4 : Sum  Inputs=+-  OutDataType=fixdt(1, 16)  OutScaling=2^0
  U1 : Outport  OutDataType=fixdt(1, 16)  OutScaling=2^0
  U2 : Outport  Port=2  OutDataType=fixdt(1, 16)  OutScaling=2^0
  U3 : Outport  Port=3  OutDataType=fixdt(1, 16)  OutScaling=2^0
  U4 : Outport  Port=4  OutDataType=fixdt(1, 16)  OutScaling=2^0
  anv_total : Outport  Port=5  OutDataType=fixdt(1, 16)  OutScaling=2^0
  wires:
  Sum/1 -> anv_total/1
  anv_prop4/1 -> Sum/4
  anv_prop3/1 -> Sum/3
  anv_prop2/1 -> Sum/2
  anv_prop1/1 -> Sum/1
  Sum1/1 -> U1/1
  F_prop1/1 -> Sum1/1, Sum3/1, Sum2/1
  F_prop2/1 -> Sum1/2, Sum4/1, Sum2/2
  F_prop3/1 -> Sum1/3, Sum3/2, Sum2/3
  F_prop4/1 -> Sum1/4, Sum4/2, Sum2/4
  l_boom/1 -> Product/2, Product1/2, Product2/2
  Sum4/1 -> Product2/1
  Sum3/1 -> Product1/1
  Sum2/1 -> Product/1
  Product2/1 -> U2/1
  Product1/1 -> U3/1
  Product/1 -> U4/1

== system Copter_Library/rate_sensor ==
  note: Sensor adds noise and Samples and quantize the Signal. In combination with the gain a integer value is generated
      | like the Sensor is read from the ADC registers.
  rate : Inport  OutDataType=fixdt(1, 16)  OutScaling=2^0
  Gain : Gain  Gain=Direction  ParameterDataType=fixdt(1, 16)  ParameterScaling=2^0  OutDataType=fixdt(1, 16)  OutScaling=2^0
  Gain20 : Gain  Gain=1/Resolution  ParameterDataType=fixdt(1, 16)  ParameterScaling=2^0  OutDataType=fixdt(1, 16)  OutScaling=2^0
  Offset : Constant  Value=Offset  OutDataType=fixdt(1, 16)  OutScaling=2^0
  Quantizer : Quantizer  QuantizationInterval=Resolution  SampleTime=Ts
  Random Number1 : RandomNumber  Variance=3.0462e-8  Seed=45632  SampleTime=0.01
  Sum : Sum  Inputs=++|  OutDataType=fixdt(1, 16)  OutScaling=2^0
  Sum14 : Sum  OutDataType=fixdt(1, 16)  OutScaling=2^0
  rate_sens : Outport  OutDataType=fixdt(1, 16)  OutScaling=2^0
  wires:
  Random Number1/1 -> Sum14/1
  Sum14/1 -> Quantizer/1
  Quantizer/1 -> Gain20/1
  rate/1 -> Sum14/2
  Offset/1 -> Sum/1
  Sum/1 -> rate_sens/1
  Gain20/1 -> Gain/1
  Gain/1 -> Sum/2

== system Copter_Library/Quadrocopter/Analysis Lab ==
  pos-vel-acc_in : Inport
  Copter Animation : Subsystem  mask(Quadrocopter Animation){AXES=[-100 100 -100 100 0 100], T_INT=1/25, K_VAR=Feste Position, K_POS=[30 0 6], K_ANGLE=27, A_ON=on, u_phi=on, u_theta=on, u_psi=on, u_x=on, u_y=on, u_z=off}
      mask prompts: AXES "Achsen Grenzen [xmin xmax ymin ymax zmin zmax]"; T_INT "Zeitintervall zwischen Aktualisierungen [s]:"; K_VAR "Kamera Art:"; K_POS "Ort der Kamera [xc yc zc]:"; K_ANGLE "Öffnungswinkel der Kamera [Grad]:"; A_ON "Animation Einschalten:"; u_phi "Use Input phi:"; u_theta "Use Input theta:"; u_psi "Use Input psi:"; u_x "Use Input x:"; u_y "Use Input y:"; u_z "Use Input z:"
      mask help: Erstellt eine 3-D animierte Ansicht eines Quadrocopters.
      mask init: same as Copter_Library/Copter Animation
      mask Help:
      | <p>Dieser Block erstellt ein 3 dimensionales Fenster eines Quadrocopters.
      | 
      | <p><H4>Block Eingänge</H4>
      | Der Eingangsvektor bestehend aus:
      | <ul>
      | <li>X-Koordinate - Ort bezogen auf die X-Achse
      | <li>Y-Koordinate - Ort bezogen auf die Y-Achse
      | <li>Z-Koordinate - Ort bezogen auf die Z-Achse
      | <li>Psi - Yaw Drehung um die Z-Achse
      | <li>Phi - Roll Drehen um die Achse in Flugrichtung
      | <li>theta - pitch Neigung in Flugrichtung nach oben bzw. unten
      | </ul></p>
      mask StyleString: edit,edit,popup(Feste Position|Frei bewegbar),edit,edit,checkbox,checkbox,checkbox,checkbox,checkbox,checkbox,checkbox
  Selector : Selector  InputPortWidth=19  IndexOptions=Index vector (dialog)  Indices=[5]  OutputSizes=1
  To File : ToFile  Filename=Record_ToFile(000)_.mat  MatrixName=Tfile
  Virtual Reality Trajectory : Subsystem
  wires:
  Selector/1 -> To File/1
  pos-vel-acc_in/1 -> Selector/1, Copter Animation/1(pos_vel_acc), Virtual Reality Trajectory/1(In1)

== system Copter_Library/Quadrocopter/Control ==
  Task : Inport  PortDimensions=4  DataType=double  OutDataTypeStr=double
  correction : Inport  Port=2
  IMU : Inport  Port=3
  height : Inport  Port=4  DataType=int16  OutDataTypeStr=int16
  Control with  optical correction or not : simulink/Signal Routing/Manual Switch  SystemSampleTime=-1  sw=1  action=0  varsize=off
  Embedded PID Control : Stateflow chart  TreatAsAtomicUnit=on
  Embedded PID Control (OC) : Stateflow chart  TreatAsAtomicUnit=on
  Embedded code  vs. Simulink Code (OC) : simulink/Signal Routing/Manual Switch  SystemSampleTime=-1  sw=0  action=0  varsize=off
  Embedded code  vs. Simulink Code : simulink/Signal Routing/Manual Switch  SystemSampleTime=-1  sw=0  action=0  varsize=off
  HIL  or Simulation : simulink/Signal Routing/Manual Switch  SystemSampleTime=-1  sw=0  action=0  varsize=off
  HIL or Simulation (OC) : simulink/Signal Routing/Manual Switch  SystemSampleTime=-1  sw=0  action=0  varsize=off
  Hardware-in-the-Loop Control : Control_lib/HIL_Control  enabled=off
  Hardware-in-the-Loop Control (OC) : Control_lib/HIL_Control  enabled=off
  Mux : Mux  Inputs=2
  Mux1 : Mux  Inputs=2
  PID_Control_IMU : Subsystem  AncestorBlock=Control_lib/PID_Regler
  PID_Control_IMU (OC) : Subsystem  AncestorBlock=Control_lib/PID_Regler
  Terminator : Terminator
  Motors : Outport  PortDimensions=4
  wires:
  IMU/1 -> Mux/1  "[ax, ay, r_phi, r_theta,r_psi]"
  Task/1 -> Mux/2  "[phi(roll), theta(pitch),rpsi(yaw rate), T(thrust)]"
  height/1 -> Terminator/1
  Control with  optical correction or not/1 -> Motors/1
  Mux/1 -> Mux1/1, PID_Control_IMU/1(u_in), Embedded PID Control/1(u), Hardware-in-the-Loop Control/1
  correction/1 -> Mux1/2  "[vx, vy, rpsi]"
  HIL  or Simulation/1 -> Control with  optical correction or not/2
  Mux1/1 -> PID_Control_IMU (OC)/1(u_in), Embedded PID Control (OC)/1(u), Hardware-in-the-Loop Control (OC)/1
  Hardware-in-the-Loop Control (OC)/1 -> Embedded code  vs. Simulink Code (OC)/2
  Embedded PID Control (OC)/1(y) -> Embedded code  vs. Simulink Code (OC)/1
  PID_Control_IMU (OC)/1(y_out) -> HIL or Simulation (OC)/1
  Embedded code  vs. Simulink Code (OC)/1 -> HIL or Simulation (OC)/2
  HIL or Simulation (OC)/1 -> Control with  optical correction or not/1
  Embedded code  vs. Simulink Code/1 -> HIL  or Simulation/1
  Hardware-in-the-Loop Control/1 -> HIL  or Simulation/2
  Embedded PID Control/1(y) -> Embedded code  vs. Simulink Code/2
  PID_Control_IMU/1(y_out) -> Embedded code  vs. Simulink Code/1

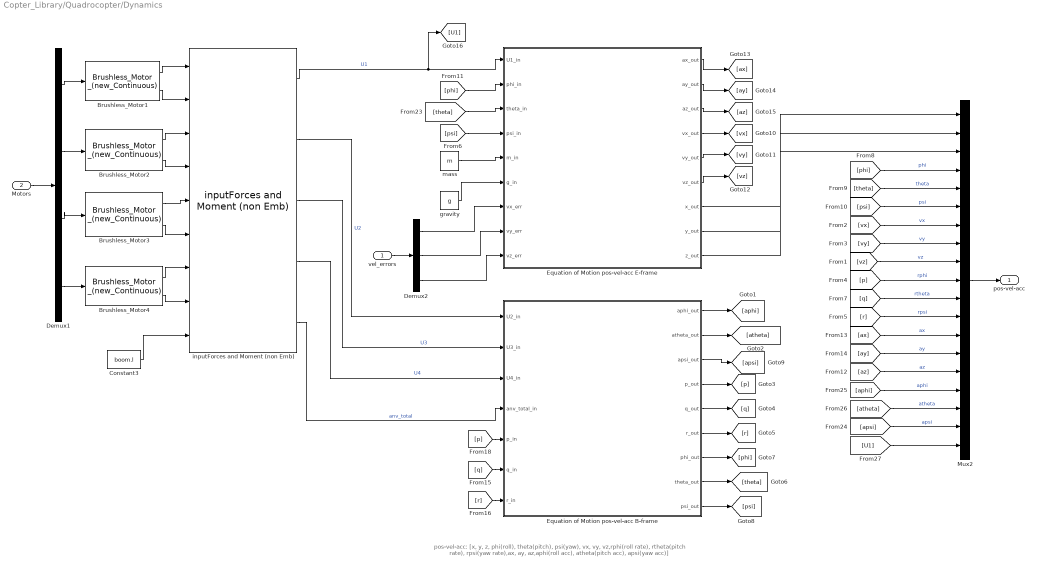
== system Copter_Library/Quadrocopter/Dynamics ==
  note: pos-vel-acc: [x, y, z, phi(roll), theta(pitch), psi(yaw), vx, vy, vz,rphi(roll rate), rtheta(pitch rate), rpsi(yaw rate),ax, ay, az,aphi(roll acc), atheta(pitch acc), apsi(yaw acc)]
  vel_errors : Inport
  Motors : Inport  Port=2
  Brushless_Motor1 : Copter_Library/Brushless_Motor _(new_Continuous)  SystemSampleTime=-1  M_error=1.01
  Brushless_Motor2 : Copter_Library/Brushless_Motor _(new_Continuous)  SystemSampleTime=-1  M_error=1.02
  Brushless_Motor3 : Copter_Library/Brushless_Motor _(new_Continuous)  SystemSampleTime=-1  M_error=0.98
  Brushless_Motor4 : Copter_Library/Brushless_Motor _(new_Continuous)  SystemSampleTime=-1  M_error=0.99
  Constant3 : Constant  Value=boom.l
  Demux1 : Demux
  Demux2 : Demux  Outputs=3
  Equation of Motion pos-vel-acc B-frame : Subsystem
  Equation of Motion pos-vel-acc E-frame : Subsystem
  Mux2 : Mux  Inputs=19
  gravity : Constant  Value=g
  inputForces and Moment (non Emb) : Copter_Library/inputForces and  Moment (non Emb)  SystemSampleTime=-1
  mass : Constant  Value=m
  pos-vel-acc : Outport
  wires:
  [apsi] -> Mux2/18  "apsi"
  [atheta] -> Mux2/17  "atheta"
  [aphi] -> Mux2/16  "aphi"
  [az] -> Mux2/15  "az"
  [ay] -> Mux2/14  "ay"
  [ax] -> Mux2/13  "ax"
  [r] -> Mux2/12  "rpsi"
  [q] -> Mux2/11  "rtheta"
  [p] -> Mux2/10  "rphi"
  [vz] -> Mux2/9  "vz"
  [vy] -> Mux2/8  "vy"
  [vx] -> Mux2/7  "vx"
  [psi] -> Mux2/6  "psi"
  [theta] -> Mux2/5  "theta"
  [phi] -> Mux2/4  "phi"
  Equation of Motion pos-vel-acc E-frame/9(z_out) -> Mux2/3
  Mux2/1 -> pos-vel-acc/1
  Motors/1 -> Demux1/1
  Demux1/3 -> Brushless_Motor3/1
  Demux1/4 -> Brushless_Motor4/1
  Demux1/2 -> Brushless_Motor2/1
  Demux1/1 -> Brushless_Motor1/1
  Constant3/1 -> inputForces and Moment (non Emb)/9
  inputForces and Moment (non Emb)/4 -> Equation of Motion pos-vel-acc B-frame/3(U4_in)  "U4"
  inputForces and Moment (non Emb)/3 -> Equation of Motion pos-vel-acc B-frame/2(U3_in)  "U3"
  inputForces and Moment (non Emb)/2 -> Equation of Motion pos-vel-acc B-frame/1(U2_in)  "U2"
  Brushless_Motor1/1 -> inputForces and Moment (non Emb)/1
  Brushless_Motor1/2 -> inputForces and Moment (non Emb)/2
  Brushless_Motor2/1 -> inputForces and Moment (non Emb)/3
  Brushless_Motor2/2 -> inputForces and Moment (non Emb)/4
  Brushless_Motor3/1 -> inputForces and Moment (non Emb)/5
  Brushless_Motor3/2 -> inputForces and Moment (non Emb)/6
  Brushless_Motor4/1 -> inputForces and Moment (non Emb)/7
  Brushless_Motor4/2 -> inputForces and Moment (non Emb)/8
  Equation of Motion pos-vel-acc E-frame/7(x_out) -> Mux2/1
  Equation of Motion pos-vel-acc E-frame/8(y_out) -> Mux2/2
  inputForces and Moment (non Emb)/1 -> [U1], Equation of Motion pos-vel-acc E-frame/1(U1_in)  "U1"
  [phi] -> Equation of Motion pos-vel-acc E-frame/2(phi_in)
  [theta] -> Equation of Motion pos-vel-acc E-frame/3(theta_in)
  [psi] -> Equation of Motion pos-vel-acc E-frame/4(psi_in)
  mass/1 -> Equation of Motion pos-vel-acc E-frame/5(m_in)
  gravity/1 -> Equation of Motion pos-vel-acc E-frame/6(g_in)
  [U1] -> Mux2/19
  Equation of Motion pos-vel-acc E-frame/4(vx_out) -> [vx]
  Equation of Motion pos-vel-acc E-frame/5(vy_out) -> [vy]
  Equation of Motion pos-vel-acc E-frame/6(vz_out) -> [vz]
  Equation of Motion pos-vel-acc E-frame/3(az_out) -> [az]
  Equation of Motion pos-vel-acc E-frame/1(ax_out) -> [ax]
  Equation of Motion pos-vel-acc E-frame/2(ay_out) -> [ay]
  inputForces and Moment (non Emb)/5 -> Equation of Motion pos-vel-acc B-frame/4(anv_total_in)  "anv_total"
  Equation of Motion pos-vel-acc B-frame/1(aphi_out) -> [aphi]
  [q] -> Equation of Motion pos-vel-acc B-frame/6(q_in)
  [r] -> Equation of Motion pos-vel-acc B-frame/7(r_in)
  [p] -> Equation of Motion pos-vel-acc B-frame/5(p_in)
  Equation of Motion pos-vel-acc B-frame/2(atheta_out) -> [atheta]
  Equation of Motion pos-vel-acc B-frame/3(apsi_out) -> [apsi]
  Equation of Motion pos-vel-acc B-frame/4(p_out) -> [p]
  Equation of Motion pos-vel-acc B-frame/5(q_out) -> [q]
  Equation of Motion pos-vel-acc B-frame/6(r_out) -> [r]
  Equation of Motion pos-vel-acc B-frame/7(phi_out) -> [phi]
  Equation of Motion pos-vel-acc B-frame/8(theta_out) -> [theta]
  Equation of Motion pos-vel-acc B-frame/9(psi_out) -> [psi]
  Demux2/1 -> Equation of Motion pos-vel-acc E-frame/7(vx_err)
  Demux2/2 -> Equation of Motion pos-vel-acc E-frame/8(vy_err)
  Demux2/3 -> Equation of Motion pos-vel-acc E-frame/9(vz_err)
  vel_errors/1 -> Demux2/1

== system Copter_Library/Quadrocopter/Environmetal influences ==
  Mux1 : Mux  Inputs=3
  Step_v_x_E_error : Step  Time=0  After=000  SampleTime=0
  Step_v_y_E_error : Step  Time=0  After=000  SampleTime=0
  Step_v_z_E_error : Step  Time=0  After=0  SampleTime=0
  vel_err : Outport
  wires:
  Mux1/1 -> vel_err/1
  Step_v_x_E_error/1 -> Mux1/1
  Step_v_y_E_error/1 -> Mux1/2
  Step_v_z_E_error/1 -> Mux1/3

== system Copter_Library/Quadrocopter/Remote Control ==
  3D-Mouse : simulink/Signal Routing/Manual Switch  SystemSampleTime=-1  sw=1  action=0  varsize=off
  Allow 3D Mouse : dspobslib/DSP Constant  SystemSampleTime=-1  Value=1  SampleMode=Discrete  discreteOutput=Sample-based  continuousOutput=Sample-based  sampTime=inf  framePeriod=2  dataType=boolean  isSigned=on  wordLen=16  udDataType=sfix(16)  fracBitsMode=Best precision  numFracBits=15  InterpretAs1D=-inf  Ts=-inf  FramebasedOutput=-inf
  Disable 3D Mouse : dspobslib/DSP Constant  SystemSampleTime=-1  Value=0  SampleMode=Discrete  discreteOutput=Sample-based  continuousOutput=Sample-based  sampTime=inf  framePeriod=2  dataType=boolean  isSigned=on  wordLen=16  udDataType=sfix(16)  fracBitsMode=Best precision  numFracBits=15  InterpretAs1D=-inf  Ts=-inf  FramebasedOutput=-inf
  Manual Switch2 : simulink/Signal Routing/Manual Switch  SystemSampleTime=-1  sw=0  action=0  varsize=off
  Remote_Control_3d_mouse : Subsystem  AncestorBlock=Remote_Control_Library/Remote_Control_3d_mouse
  Remote_Control_Pitch_stimuli1 : Subsystem  AncestorBlock=Remote_Control_Library/Remote_Control_Pitch_stimuli
  RC_out : Outport
  wires:
  Remote_Control_Pitch_stimuli1/1(Out) -> Manual Switch2/1
  Manual Switch2/1 -> RC_out/1
  Allow 3D Mouse/1 -> 3D-Mouse/1
  Disable 3D Mouse/1 -> 3D-Mouse/2
  3D-Mouse/1 -> Remote_Control_3d_mouse/Enable
  Remote_Control_3d_mouse/1(Out1) -> Manual Switch2/2

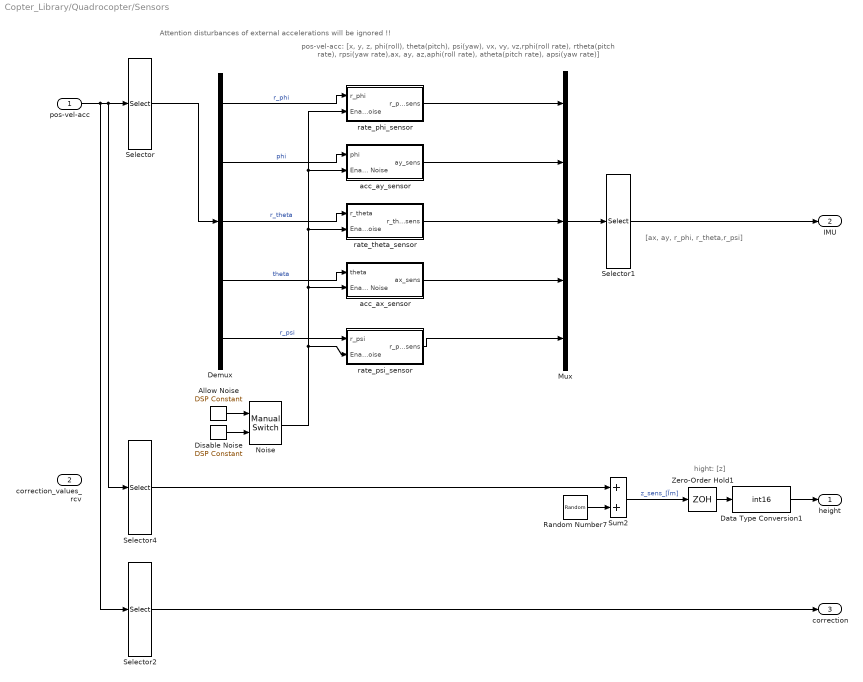
== system Copter_Library/Quadrocopter/Sensors ==
  note: Attention disturbances of external accelerations will be ignored !!
  note: hight: [z]
  note: pos-vel-acc: [x, y, z, phi(roll), theta(pitch), psi(yaw), vx, vy, vz,rphi(roll rate), rtheta(pitch rate), rpsi(yaw rate),ax, ay, az,aphi(roll rate), atheta(pitch rate), apsi(yaw rate)]
  note: [ax, ay, r_phi, r_theta,r_psi]
  pos-vel-acc : Inport  PortDimensions=19
  correction_values_rcv : Inport  Port=2  PortDimensions=19
  Allow Noise : dspobslib/DSP Constant  SystemSampleTime=-1  Value=1  SampleMode=Discrete  discreteOutput=Sample-based  continuousOutput=Sample-based  sampTime=inf  framePeriod=2  dataType=boolean  isSigned=on  wordLen=16  udDataType=sfix(16)  fracBitsMode=Best precision  numFracBits=15  InterpretAs1D=-inf  Ts=-inf  FramebasedOutput=-inf
  Data Type Conversion1 : DataTypeConversion  OutDataTypeMode=int16  OutDataTypeStr=int16  RndMeth=Round
  Demux : Demux  Outputs=5
  Disable Noise : dspobslib/DSP Constant  SystemSampleTime=-1  Value=0  SampleMode=Discrete  discreteOutput=Sample-based  continuousOutput=Sample-based  sampTime=inf  framePeriod=2  dataType=boolean  isSigned=on  wordLen=16  udDataType=sfix(16)  fracBitsMode=Best precision  numFracBits=15  InterpretAs1D=-inf  Ts=-inf  FramebasedOutput=-inf
  Mux : Mux  Inputs=5
  Noise : simulink/Signal Routing/Manual Switch  SystemSampleTime=-1  sw=1  action=0  varsize=off
  Random Number7 : RandomNumber  Variance=3.0462e-8  Seed=5756  SampleTime=0.01
  Selector : Selector  InputPortWidth=19  IndexOptions=Index vector (dialog)  Indices=[10 4 11 5 12]  OutputSizes=1
  Selector1 : Selector  InputPortWidth=5  IndexOptions=Index vector (dialog)  Indices=[4 2 1 3 5]  OutputSizes=1
  Selector2 : Selector  InputPortWidth=19  IndexOptions=Index vector (dialog)  Indices=[7 8 12]  OutputSizes=1
  Selector4 : Selector  InputPortWidth=19  IndexOptions=Index vector (dialog)  Indices=[3]  OutputSizes=1
  Sum2 : Sum
  Zero-Order Hold1 : ZeroOrderHold  SampleTime=Ts
  acc_ax_sensor : Subsystem
  acc_ay_sensor : Subsystem
  rate_phi_sensor : Subsystem
  rate_psi_sensor : Subsystem
  rate_theta_sensor : Subsystem
  height : Outport
  IMU : Outport  Port=2
  correction : Outport  Port=3
  wires:
  pos-vel-acc/1 -> Selector2/1, Selector/1, Selector4/1
  Selector/1 -> Demux/1
  rate_phi_sensor/1(r_phi_sens) -> Mux/1
  acc_ay_sensor/1(ay_sens) -> Mux/2
  rate_theta_sensor/1(r_theta_sens) -> Mux/3
  acc_ax_sensor/1(ax_sens) -> Mux/4
  rate_psi_sensor/1(r_psi_sens) -> Mux/5
  Demux/1 -> rate_phi_sensor/1(r_phi)  "r_phi"
  Demux/2 -> acc_ay_sensor/1(phi)  "phi"
  Demux/3 -> rate_theta_sensor/1(r_theta)  "r_theta"
  Demux/4 -> acc_ax_sensor/1(theta)  "theta"
  Demux/5 -> rate_psi_sensor/1(r_psi)  "r_psi"
  Mux/1 -> Selector1/1
  Selector1/1 -> IMU/1
  Allow Noise/1 -> Noise/1
  Disable Noise/1 -> Noise/2
  Noise/1 -> rate_psi_sensor/2(Enable Noise), acc_ax_sensor/2(Enable Noise), rate_theta_sensor/2(Enable Noise), acc_ay_sensor/2(Enable Noise), rate_phi_sensor/2(Enable Noise)
  Random Number7/1 -> Sum2/2
  Selector4/1 -> Sum2/1
  Sum2/1 -> Zero-Order Hold1/1  "z_sens_[Ïm]"
  Zero-Order Hold1/1 -> Data Type Conversion1/1
  Data Type Conversion1/1 -> height/1
  Selector2/1 -> correction/1

== system Copter_Library/Quadrocopter/Analysis Lab/Copter Animation ==
  pos_vel_acc : Inport  PortDimensions=19
  S-Function : S-Function  FunctionName=Copter_Animation  Parameters=Config  EnableBusSupport=off
  Selector2 : Selector  InputPortWidth=19  IndexOptions=Index vector (dialog)  Indices=[1 2 3 4 5 6]  OutputSizes=1
  wires:
  pos_vel_acc/1 -> Selector2/1
  Selector2/1 -> S-Function/1

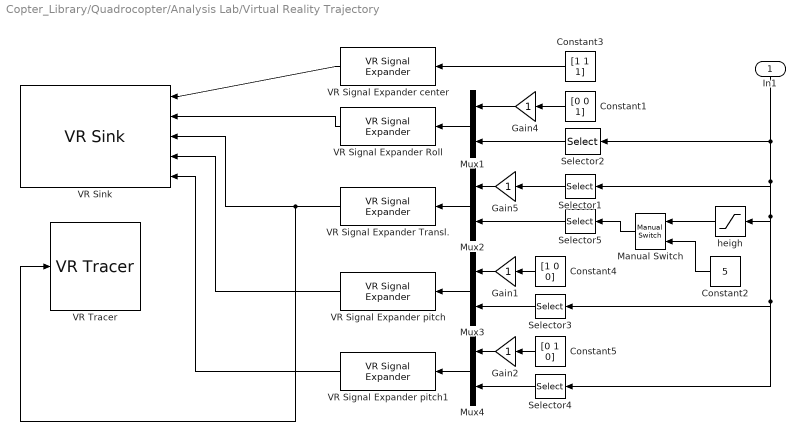
== system Copter_Library/Quadrocopter/Analysis Lab/Virtual Reality Trajectory ==
  In1 : Inport
  Constant1 : Constant  Value=[0 0 1]
  Constant2 : Constant  Value=5
  Constant3 : Constant  Value=[1 1 1]
  Constant4 : Constant  Value=[1 0 0]
  Constant5 : Constant  Value=[0 1 0]
  Gain{1..2,4..5} (4 alike) : Gain  ParameterDataType=fixdt(1, 16)  ParameterScaling=2^0  OutDataType=fixdt(1, 16)  OutScaling=2^0
  Manual Switch : simulink/Signal Routing/Manual Switch  SystemSampleTime=-1  sw=0  action=0  varsize=off
  Mux{1..4} (4 alike) : Mux  Inputs=2
  Selector1 : Selector  InputPortWidth=19  IndexOptions=Index vector (dialog)  Indices=[1 2]  OutputSizes=1
  Selector2 : Selector  InputPortWidth=19  IndexOptions=Index vector (dialog)  Indices=[4]  OutputSizes=1
  Selector3 : Selector  InputPortWidth=19  IndexOptions=Index vector (dialog)  Indices=[5]  OutputSizes=1
  Selector4 : Selector  InputPortWidth=19  IndexOptions=Index vector (dialog)  Indices=[6]  OutputSizes=1
  Selector5 : Selector  InputPortWidth=19  IndexOptions=Index vector (dialog)  Indices=[3]  OutputSizes=1
  VR Signal Expander Roll : vrlib/VR Signal Expander  SystemSampleTime=-1  outwidth=4  outidx=[1 2 3 4]
  VR Signal Expander Transl. : vrlib/VR Signal Expander  SystemSampleTime=-1  outwidth=3  outidx=[3 1 2]
  VR Signal Expander center : vrlib/VR Signal Expander  SystemSampleTime=-1  outwidth=3  outidx=[1 2 3]
  VR Signal Expander pitch : vrlib/VR Signal Expander  SystemSampleTime=-1  outwidth=4  outidx=[1 2 3 4]
  VR Signal Expander pitch1 : vrlib/VR Signal Expander  SystemSampleTime=-1  outwidth=4  outidx=[1 2 3 4]
  VR Sink : vrlib/VR Sink  InstantiateOnLoad=on  SampleTime=0.1  ViewEnable=on  RemoteChange=off  RemoteView=off  FieldsWritten=Roll_Trans.center.3.1.1.double#Roll_Trans.rotation.4.1.1.double#Roll_Trans.translation.3.1.1.double#Pitch_Trans.rotation.4.1.1.double#Yaw_Trans.rotation.4.1.1.double  WorldFileName=VRML1.WRL  AutoView=on  VideoDimensions=[]
  VR Tracer : vrlib/VR Tracer  VrmlFile=VRML1.WRL  ParentNode=Ground  MarkerName=None  UseLines=on  UseTriads=on  MarkerScale=[1 1 1]  MarkerColorSelection=Defined as RGB values  MarkerColor=red  rgbval=[1 0 0]  Ts=1  ForceViewerOpen=off
  heigh : Saturate  UpperLimit=inf  LowerLimit=0  OutDataType=fixdt(1, 16)  OutScaling=2^0
  wires:
  Selector1/1 -> Gain5/1
  Constant1/1 -> Gain4/1
  Selector2/1 -> Mux1/2
  Mux1/1 -> VR Signal Expander Roll/1
  Constant3/1 -> VR Signal Expander center/1
  VR Signal Expander center/1 -> VR Sink/1
  VR Signal Expander Roll/1 -> VR Sink/2
  VR Signal Expander Transl./1 -> VR Sink/3, VR Tracer/1
  Mux2/1 -> VR Signal Expander Transl./1
  Mux3/1 -> VR Signal Expander pitch/1
  Selector3/1 -> Mux3/2
  Constant4/1 -> Gain1/1
  VR Signal Expander pitch/1 -> VR Sink/4
  Mux4/1 -> VR Signal Expander pitch1/1
  Selector4/1 -> Mux4/2
  Constant5/1 -> Gain2/1
  VR Signal Expander pitch1/1 -> VR Sink/5
  Gain5/1 -> Mux2/1
  Gain1/1 -> Mux3/1
  Gain2/1 -> Mux4/1
  Gain4/1 -> Mux1/1
  In1/1 -> Selector2/1, Selector1/1, Selector3/1, Selector4/1, heigh/1
  Selector5/1 -> Mux2/2
  heigh/1 -> Manual Switch/1
  Constant2/1 -> Manual Switch/2
  Manual Switch/1 -> Selector5/1
